simulink model "CODE_GEN"  (R2023b)
settings: Solver=FixedStepDiscrete  StartTime=0.0  StopTime=10.0  FixedStep=0.001  RelTol=1e-3
undefined symbols (not defined in the file): E_up, eta, g, I, k_cw, k_em, k_lqr, k_su, k_vw, L, m, uMax, x1_max, x2_max
settings Model: Creator=doann  LastModifiedBy=doann
settings OptimizationCC: DefaultParameterBehavior=Inlined  UseDivisionForNetSlopeComputation=on  GainParamInheritBuiltInType=on  UseFloatMulNetSlope=on  InlineInvariantSignals=on  PassReuseOutputArgsAs=Individual arguments  ZeroExternalMemoryAtStartup=off  ZeroInternalMemoryAtStartup=off  NoFixptDivByZeroProtection=on  EfficientFloat2IntCast=on  LifeSpan=1  OptimizeBlockOrder=speed  DifferentSizesBufferReuse=on  EfficientTunableParamExpr=on
settings DebuggingCC: ParameterTunabilityLossMsg=error
settings HardwareCC: ProdBitPerPointer=32  ProdBitPerSizeT=32  ProdBitPerPtrDiffT=32  ProdLargestAtomicInteger=Long  ProdLargestAtomicFloat=Double  ProdWordSize=32  ProdLongLongMode=on  ProdHWDeviceType=ARM Compatible->ARM Cortex-M
settings SFSimCC: MATLABDynamicMemAlloc=off
settings RTWCC: Description=Embedded Coder  SystemTargetFile=ert.tlc  TemplateMakefile=ert_default_tmf  TargetLang=C++
settings CodeAppCC: ForceParamTrailComments=on  IgnoreCustomStorageClasses=off  OperatorAnnotations=on  SimulinkDataObjDesc=on  SFDataObjDesc=on  CustomSymbolStrGlobalVar=rt$N$M  CustomSymbolStrType=$N$M  CustomSymbolStrFcn=$N$M$F  CustomSymbolStrMacro=$N$M  InsertBlockDesc=on
settings ERTTargetCC: TargetLangStandard=C++11 (ISO)  GenerateSampleERTMain=on  IncludeMdlTerminateFcn=off  CombineSignalStateStructs=on  SupportAbsoluteTime=off  CodeInterfacePackaging=C++ class  SupportComplex=off  SupportNonInlinedSFcns=on  InlinedParameterPlacement=NonHierarchical  RootIOFormat=Structure reference  ERTCustomFileTemplate=example_file_process.tlc  ERTFilePackagingFormat=CompactWithDataFile

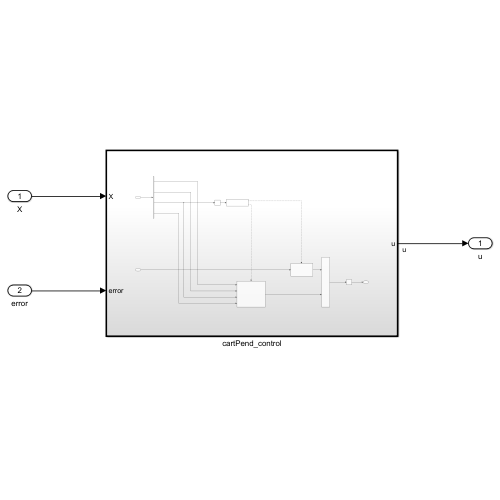
[thumbnail: Simulink's stored preview of the top-level diagram]
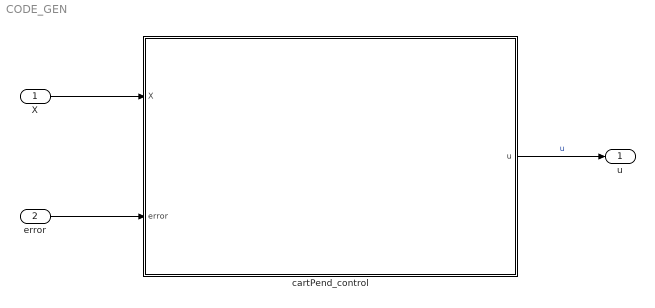
== system CODE_GEN ==
  X : Inport
  error : Inport  Port=2
  cartPend_control : Subsystem  TreatAsAtomicUnit=on  SystemSampleTime=0.001
  u : Outport
  wires:
  cartPend_control/1(u) -> u/1  "u"
  X/1 -> cartPend_control/1(X)
  error/1 -> cartPend_control/2(error)

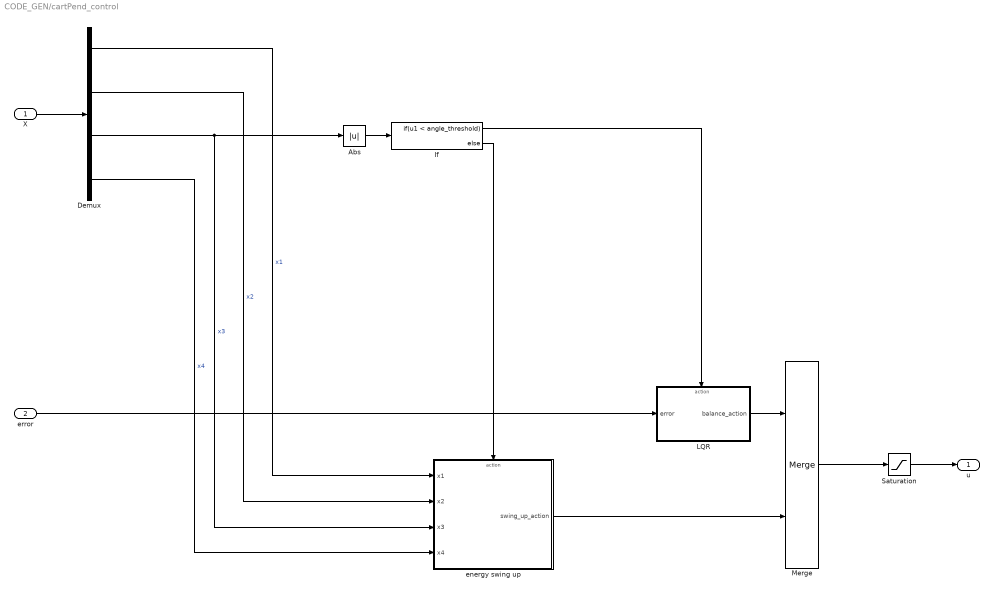
== system CODE_GEN/cartPend_control ==
  X : Inport
  error : Inport  Port=2
  Abs : Abs  SaturateOnIntegerOverflow=off
  Demux : Demux
  If : If  IfExpression=u1 < angle_threshold
  LQR : Subsystem  TreatAsAtomicUnit=on
  Merge : Merge
  Saturation : Saturate  UpperLimit=uMax  LowerLimit=-uMax
  energy swing up : Subsystem  TreatAsAtomicUnit=on
  u : Outport
  wires:
  X/1 -> Demux/1
  Demux/3 -> Abs/1, energy swing up/3(x3)  "x3"
  Demux/4 -> energy swing up/4(x4)  "x4"
  Abs/1 -> If/1
  If/1 -> LQR/Action
  If/2 -> energy swing up/Action
  LQR/1(balance_action) -> Merge/1
  energy swing up/1(swing_up_action) -> Merge/2
  error/1 -> LQR/1(error)
  Demux/2 -> energy swing up/2(x2)  "x2"
  Demux/1 -> energy swing up/1(x1)  "x1"
  Merge/1 -> Saturation/1
  Saturation/1 -> u/1

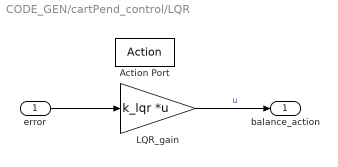
== system CODE_GEN/cartPend_control/LQR ==
  error : Inport
  Action Port : ActionPort  ActionPortLabel=if(u1 < angle_threshold)
  LQR_gain : Gain  Gain=k_lqr  Multiplication=Matrix(K*u)
  balance_action : Outport
  wires:
  error/1 -> LQR_gain/1
  LQR_gain/1 -> balance_action/1  "u"

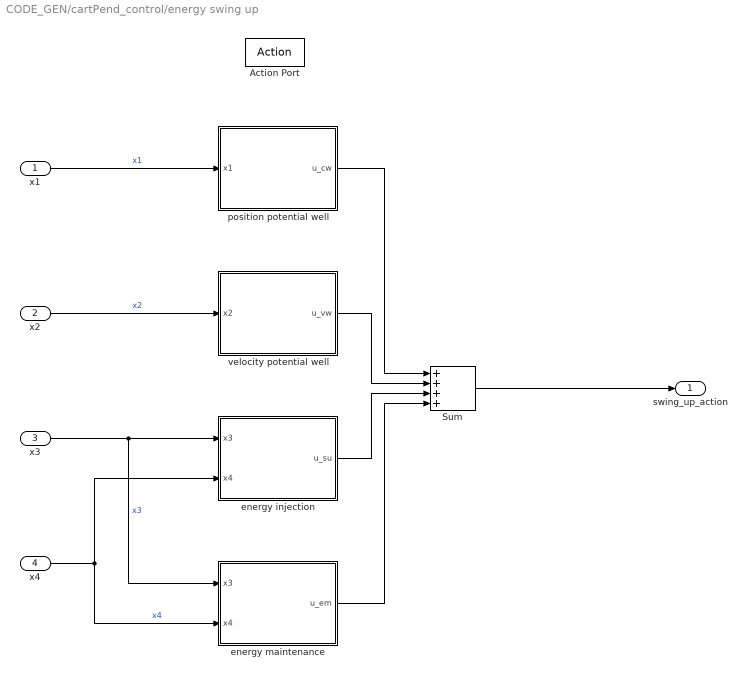
== system CODE_GEN/cartPend_control/energy swing up ==
  x1 : Inport
  x2 : Inport  Port=2
  x3 : Inport  Port=3
  x4 : Inport  Port=4
  Action Port : ActionPort  ActionPortLabel=else
  Sum : Sum  Inputs=++++
  energy injection : Subsystem
  energy maintenance : Subsystem
  position potential well : Subsystem
  velocity potential well : Subsystem
  swing_up_action : Outport
  wires:
  energy injection/1(u_su) -> Sum/3
  x2/1 -> velocity potential well/1(x2)  "x2"
  velocity potential well/1(u_vw) -> Sum/2
  Sum/1 -> swing_up_action/1
  energy maintenance/1(u_em) -> Sum/4
  x3/1 -> energy maintenance/1(x3), energy injection/1(x3)  "x3"
  x1/1 -> position potential well/1(x1)  "x1"
  x4/1 -> energy injection/2(x4), energy maintenance/2(x4)  "x4"
  position potential well/1(u_cw) -> Sum/1

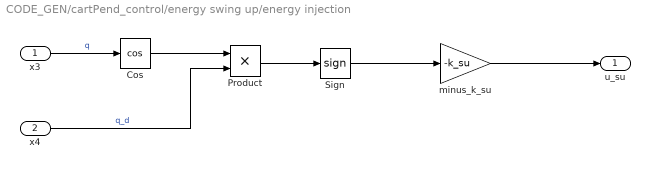
== system CODE_GEN/cartPend_control/energy swing up/energy injection ==
  x3 : Inport
  x4 : Inport  Port=2
  Cos : Trigonometry  Operator=cos
  Product : Product
  Sign : Signum
  minus_k_su : Gain  Gain=-k_su
  u_su : Outport
  wires:
  x3/1 -> Cos/1  "q"
  x4/1 -> Product/2  "q_d"
  Sign/1 -> minus_k_su/1
  minus_k_su/1 -> u_su/1
  Cos/1 -> Product/1
  Product/1 -> Sign/1

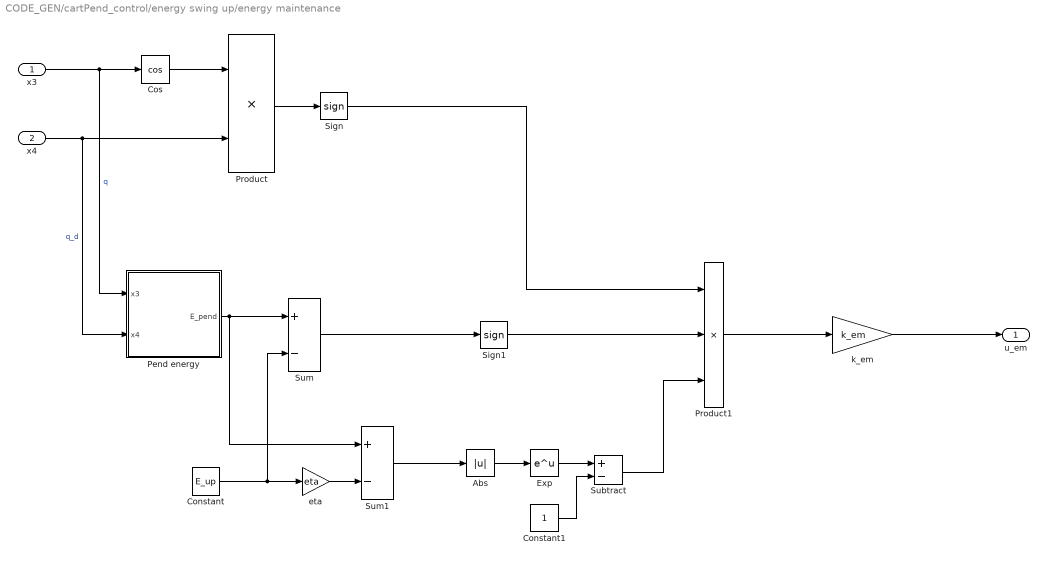
== system CODE_GEN/cartPend_control/energy swing up/energy maintenance ==
  x3 : Inport
  x4 : Inport  Port=2
  Abs : Abs  SaturateOnIntegerOverflow=off
  Constant : Constant  Value=E_up
  Constant1 : Constant
  Cos : Trigonometry  Operator=cos
  Exp : Math
  Pend energy : Subsystem
  Product : Product
  Product1 : Product  Inputs=3
  Sign : Signum
  Sign1 : Signum
  Subtract : Sum  Inputs=+-
  Sum : Sum  Inputs=+-
  Sum1 : Sum  Inputs=+-
  eta : Gain  Gain=eta
  k_em : Gain  Gain=k_em
  u_em : Outport
  wires:
  x3/1 -> Pend energy/1(x3), Cos/1  "q"
  Cos/1 -> Product/1
  x4/1 -> Pend energy/2(x4), Product/2  "q_d"
  Product/1 -> Sign/1
  Pend energy/1(E_pend) -> Sum/1, Sum1/1
  Constant/1 -> Sum/2, eta/1
  Sum/1 -> Sign1/1
  eta/1 -> Sum1/2
  Sum1/1 -> Abs/1
  Abs/1 -> Exp/1
  Exp/1 -> Subtract/1
  Constant1/1 -> Subtract/2
  Sign1/1 -> Product1/2
  Sign/1 -> Product1/1
  Subtract/1 -> Product1/3
  Product1/1 -> k_em/1
  k_em/1 -> u_em/1

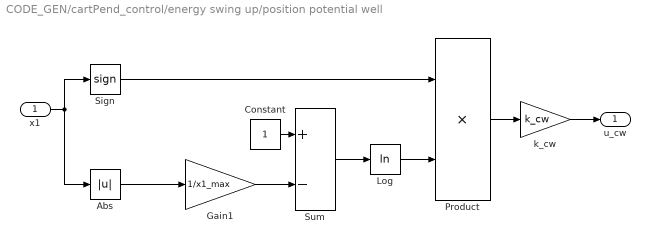
== system CODE_GEN/cartPend_control/energy swing up/position potential well ==
  x1 : Inport
  Abs : Abs  SaturateOnIntegerOverflow=off
  Constant : Constant
  Gain1 : Gain  Gain=1/x1_max
  Log : Math  Operator=log
  Product : Product
  Sign : Signum
  Sum : Sum  Inputs=+-
  k_cw : Gain  Gain=k_cw
  u_cw : Outport
  wires:
  x1/1 -> Abs/1, Sign/1
  Abs/1 -> Gain1/1
  Gain1/1 -> Sum/2
  Constant/1 -> Sum/1
  Sum/1 -> Log/1
  k_cw/1 -> u_cw/1
  Product/1 -> k_cw/1
  Log/1 -> Product/2
  Sign/1 -> Product/1

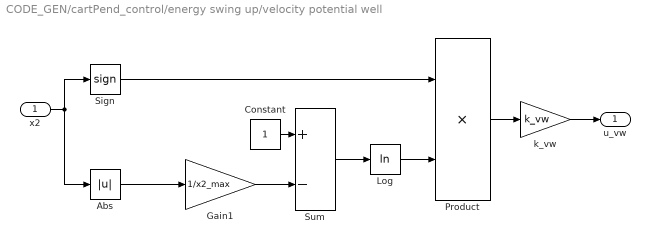
== system CODE_GEN/cartPend_control/energy swing up/velocity potential well ==
  x2 : Inport
  Abs : Abs  SaturateOnIntegerOverflow=off
  Constant : Constant
  Gain1 : Gain  Gain=1/x2_max
  Log : Math  Operator=log
  Product : Product
  Sign : Signum
  Sum : Sum  Inputs=+-
  k_vw : Gain  Gain=k_vw
  u_vw : Outport
  wires:
  Sign/1 -> Product/1
  Log/1 -> Product/2
  Product/1 -> k_vw/1
  k_vw/1 -> u_vw/1
  Sum/1 -> Log/1
  Constant/1 -> Sum/1
  Gain1/1 -> Sum/2
  Abs/1 -> Gain1/1
  x2/1 -> Sign/1, Abs/1

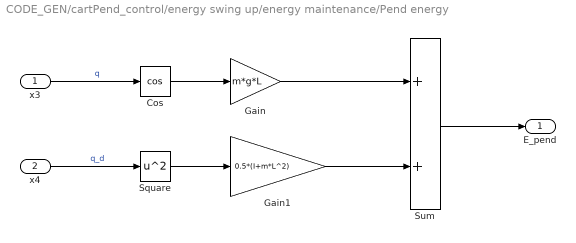
== system CODE_GEN/cartPend_control/energy swing up/energy maintenance/Pend energy ==
  x3 : Inport
  x4 : Inport  Port=2
  Cos : Trigonometry  Operator=cos
  Gain : Gain  Gain=m*g*L
  Gain1 : Gain  Gain=0.5*(I+m*L^2)
  Square : Math  Operator=square
  Sum : Sum
  E_pend : Outport
  wires:
  x3/1 -> Cos/1  "q"
  x4/1 -> Square/1  "q_d"
  Cos/1 -> Gain/1
  Square/1 -> Gain1/1
  Gain/1 -> Sum/1
  Gain1/1 -> Sum/2
  Sum/1 -> E_pend/1
